simulink model "BLOM_ex"  (Simulink 7.4)
settings: Solver=FixedStepDiscrete  StartTime=0.0  StopTime=40  FixedStep=1  RelTol=1e-3
undefined symbols (not defined in the file or in its folder): AR_A, AR_C, mix_A, mix_C, x1, x2
libraries: MPCMdlLib x34
settings Model: Creator=vichik  LastModifiedBy=sergv
settings OptimizationCC: InitFltsAndDblsToZero=on

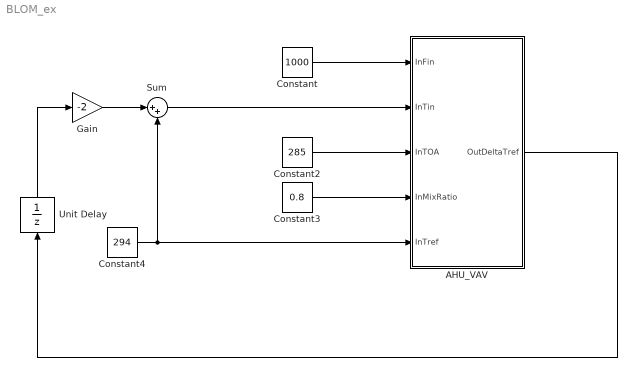
== system BLOM_ex ==
  AHU_VAV : Subsystem
  Constant : Constant  Value=1000  OutDataType=sfix(16)  OutScaling=2^0
  Constant2 : Constant  Value=285  OutDataType=sfix(16)  OutScaling=2^0
  Constant3 : Constant  Value=0.8  OutDataType=sfix(16)  OutScaling=2^0
  Constant4 : Constant  Value=294  OutDataType=sfix(16)  OutScaling=2^0
  Gain : Gain  Gain=-2  ParameterDataType=sfix(16)  ParameterScaling=2^0  OutDataType=sfix(16)  OutScaling=2^0
  Sum : Sum  Inputs=|++  OutDataType=sfix(16)  OutScaling=2^0
  Unit Delay : UnitDelay  SampleTime=-1
  wires:
  Constant/1 -> AHU_VAV/1(InFin)
  Constant2/1 -> AHU_VAV/3(InTOA)
  Constant3/1 -> AHU_VAV/4(InMixRatio)
  Constant4/1 -> Sum/2, AHU_VAV/5(InTref)
  Sum/1 -> AHU_VAV/2(InTin)
  Gain/1 -> Sum/1
  Unit Delay/1 -> Gain/1
  AHU_VAV/1(OutDeltaTref) -> Unit Delay/1

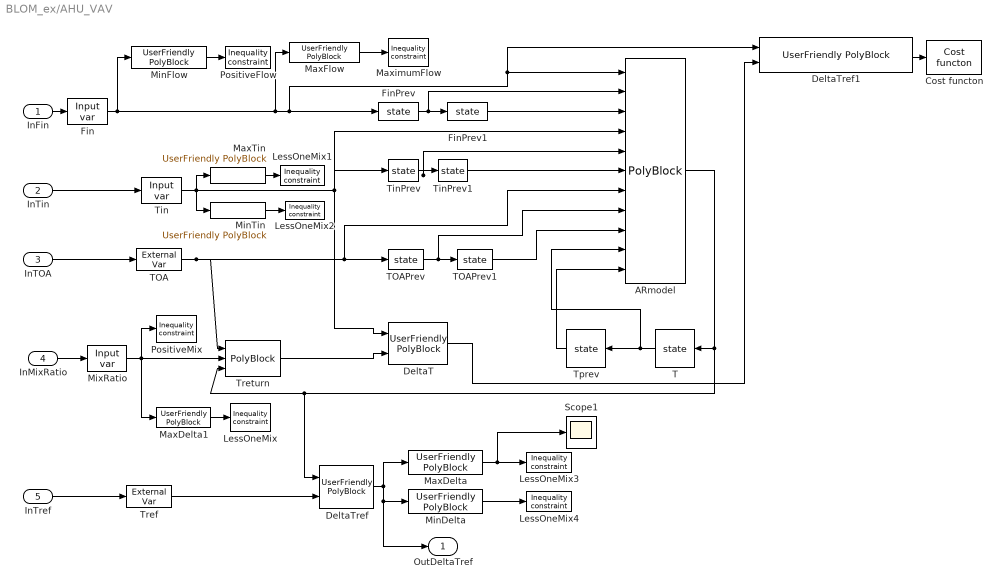
== system BLOM_ex/AHU_VAV ==
  InFin : Inport
  InTin : Inport  Port=2
  InTOA : Inport  Port=3
  InMixRatio : Inport  Port=4
  InTref : Inport  Port=5
  ARmodel : MPCMdlLib/PolyBlock  Tag=PolyBlock  A=AR_A  C=AR_C  input_type=Scalar  output_type=Scalar
  Cost functon : MPCMdlLib/Cost functon  Tag=OptCost
  DeltaT : MPCMdlLib/UserFriendly PolyBlock  Tag=PolyBlock  A="[1  0  ; 0 1 ]"  C="[1  -1]"  gA=[0 0]  gC=1  input_type=Scalar  output_type=Scalar  port_names=x1,x2
  DeltaTref : MPCMdlLib/UserFriendly PolyBlock  Tag=PolyBlock  A="[1  0  ; 0 1 ]"  C="[1  -1]"  gA=[0 0]  gC=1  input_type=Scalar  output_type=Scalar  port_names=x1,x2
  DeltaTref1 : MPCMdlLib/UserFriendly PolyBlock  Tag=PolyBlock  A="[2  0  ; 0 2 ]"  C=[0.00001 1]  gA=[0 0]  gC=1  input_type=Scalar  output_type=Scalar  port_names=x1,x2
  Fin : MPCMdlLib/Input var  Tag=OptInput  SystemSampleTime=-1  step_ratio=1  save_name=AHU_VAV_Fin
  FinPrev : MPCMdlLib/state  Tag=OptState  SystemSampleTime=-1  init_val=1000  save_name=AHU_VAV_FinPrev
  FinPrev1 : MPCMdlLib/state  Tag=OptState  SystemSampleTime=-1  init_val=1000  save_name=AHU_VAV_FinPrev1
  LessOneMix{,1..4} (5 alike) : MPCMdlLib/Inequality constraint  Tag=InequalBlock  CompareSign=> 0
  MaxDelta : MPCMdlLib/UserFriendly PolyBlock  Tag=PolyBlock  A="[0  ;1]"  C=[2 -1]  gA=[0 ]  gC=1  input_type=Scalar  output_type=Scalar  port_names=u
  MaxDelta1 : MPCMdlLib/UserFriendly PolyBlock  Tag=PolyBlock  A="[0  ;1]"  C=[1 -1]  gA=[0 ]  gC=1  input_type=Scalar  output_type=Scalar  port_names=x1,x2
  MaxFlow : MPCMdlLib/UserFriendly PolyBlock  Tag=PolyBlock  A="[0  ; 1]"  C=[4000 -1]  gA=[0 ]  gC=1  input_type=Scalar  output_type=Scalar  port_names=x1,x2
  MaxTin : MPCMdlLib/UserFriendly PolyBlock  Tag=PolyBlock  A="[0  ; 1]"  C=[310 -1]  gA=[0 ]  gC=1  input_type=Scalar  output_type=Scalar  port_names=x1,x2
  MaximumFlow : MPCMdlLib/Inequality constraint  Tag=InequalBlock  CompareSign=> 0
  MinDelta : MPCMdlLib/UserFriendly PolyBlock  Tag=PolyBlock  A="[1  ; 0]"  C=[1 2]  gA=[0 ]  gC=1  input_type=Scalar  output_type=Scalar  port_names=x1,x2
  MinFlow : MPCMdlLib/UserFriendly PolyBlock  Tag=PolyBlock  A="[1  ; 0]"  C=[1 -50]  gA=[0 ]  gC=1  input_type=Scalar  output_type=Scalar  port_names=x1,x2
  MinTin : MPCMdlLib/UserFriendly PolyBlock  Tag=PolyBlock  A="[1  ; 0]"  C=[1 -260]  gA=[0 ]  gC=1  input_type=Scalar  output_type=Scalar  port_names=x1,x2
  MixRatio : MPCMdlLib/Input var  Tag=OptInput  SystemSampleTime=-1  step_ratio=1  save_name=AHU_VAV_MixRatio
  PositiveFlow : MPCMdlLib/Inequality constraint  Tag=InequalBlock  CompareSign=> 0
  PositiveMix : MPCMdlLib/Inequality constraint  Tag=InequalBlock  CompareSign=> 0
  Scope1 : Scope
      settings: TimeRange=10
  T : MPCMdlLib/state  Tag=OptState  SystemSampleTime=-1  init_val=293  save_name=AHU_VAV_T
  TOA : MPCMdlLib/External Var  Tag=OptExternal  SystemSampleTime=-1  save_name=AHU_VAV_TOA
  TOAPrev : MPCMdlLib/state  Tag=OptState  SystemSampleTime=-1  init_val=285  save_name=AHU_VAV_TOAPrev
  TOAPrev1 : MPCMdlLib/state  Tag=OptState  SystemSampleTime=-1  init_val=285  save_name=AHU_VAV_TOAPrev1
  Tin : MPCMdlLib/Input var  Tag=OptInput  SystemSampleTime=-1  step_ratio=1  save_name=AHU_VAV_Tin
  TinPrev : MPCMdlLib/state  Tag=OptState  SystemSampleTime=-1  init_val=294  save_name=AHU_VAV_TinPrev
  TinPrev1 : MPCMdlLib/state  Tag=OptState  SystemSampleTime=-1  init_val=294  save_name=AHU_VAV_TinPrev1
  Tprev : MPCMdlLib/state  Tag=OptState  SystemSampleTime=-1  init_val=293  save_name=AHU_VAV_Tprev
  Tref : MPCMdlLib/External Var  Tag=OptExternal  SystemSampleTime=-1  save_name=AHU_VAV_Tref
  Treturn : MPCMdlLib/PolyBlock  Tag=PolyBlock  A=mix_A  C=mix_C  input_type=Scalar  output_type=Scalar
  OutDeltaTref : Outport
  wires:
  Fin/1 -> FinPrev/1, DeltaTref1/1, ARmodel/1, MaxFlow/1, MinFlow/1
  Tin/1 -> TinPrev/1, ARmodel/4, DeltaT/1, MinTin/1, MaxTin/1
  FinPrev/1 -> FinPrev1/1, ARmodel/2
  TOA/1 -> Treturn/1, TOAPrev/1, ARmodel/7
  MaxFlow/1 -> MaximumFlow/1
  MixRatio/1 -> PositiveMix/1, MaxDelta1/1, Treturn/2
  MaxDelta1/1 -> LessOneMix/1
  MaxTin/1 -> LessOneMix1/1
  MinTin/1 -> LessOneMix2/1
  T/1 -> Tprev/1, ARmodel/10
  ARmodel/1 -> T/1, DeltaTref/1, Treturn/3
  Tref/1 -> DeltaTref/2
  DeltaTref/1 -> MinDelta/1, OutDeltaTref/1, MaxDelta/1
  DeltaT/1 -> DeltaTref1/2
  DeltaTref1/1 -> Cost functon/1
  TinPrev/1 -> TinPrev1/1, ARmodel/5
  FinPrev1/1 -> ARmodel/3
  TinPrev1/1 -> ARmodel/6
  TOAPrev/1 -> TOAPrev1/1, ARmodel/8
  TOAPrev1/1 -> ARmodel/9
  Tprev/1 -> ARmodel/11
  MinFlow/1 -> PositiveFlow/1
  MinDelta/1 -> LessOneMix4/1
  MaxDelta/1 -> LessOneMix3/1, Scope1/1
  InTref/1 -> Tref/1
  InFin/1 -> Fin/1
  InTin/1 -> Tin/1
  InTOA/1 -> TOA/1
  InMixRatio/1 -> MixRatio/1
  Treturn/1 -> DeltaT/2
